simulink model "extTorqueObserver"  (R2017b)
settings: Solver=VariableStepAuto  StartTime=0.0  StopTime=10.0  RelTol=1e-3
undefined symbols (not defined in the file): D, Denv, F, g_reac, I, J_inv, Jmn, Jn, Kenv, Kt, Ktn, M, s, tau_g, tau_int
settings Model: Creator=dinies33  LastModifiedBy=dinies33

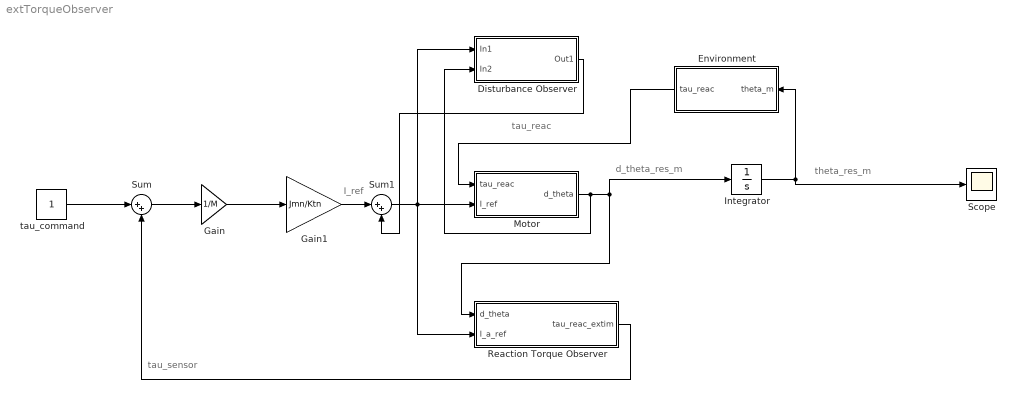
== system extTorqueObserver ==
  note: tau_sensor
  note: tau_reac
  note: theta_res_m
  note: d_theta_res_m
  note: I_ref
  Disturbance Observer : Subsystem
  Environment : Subsystem
  Gain : Gain  Gain=1/M
  Gain1 : Gain  Gain=Jmn/Ktn
  Integrator : Integrator
  Motor : Subsystem
  "Reaction Torque Observer " : Subsystem
  Scope : Scope
  Sum : Sum  Inputs=|++
  Sum1 : Sum  Inputs=|++
  "tau_command " : Constant
  wires:
  Sum/1 -> Gain/1
  Gain/1 -> Gain1/1
  Gain1/1 -> Sum1/1
  Sum1/1 -> Disturbance Observer/1(In1), Motor/2(I_ref), "Reaction Torque Observer "/2("I_a_ref ")
  Motor/1("d_theta ") -> "Reaction Torque Observer "/1("d_theta "), Integrator/1, Disturbance Observer/2(In2)
  Disturbance Observer/1(Out1) -> Sum1/2
  "Reaction Torque Observer "/1("tau_reac_extim ") -> Sum/2
  Environment/1("tau_reac ") -> Motor/1(tau_reac)
  Integrator/1 -> Scope/1, Environment/1(theta_m)
  "tau_command "/1 -> Sum/1

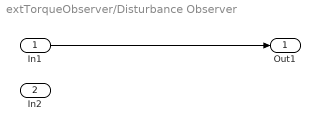
== system extTorqueObserver/Disturbance Observer ==
  In1 : Inport
  In2 : Inport  Port=2
  Out1 : Outport
  wires:
  In1/1 -> Out1/1

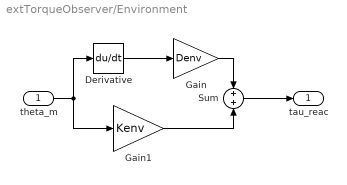
== system extTorqueObserver/Environment ==
  theta_m : Inport
  Derivative : Derivative  CoefficientInTFapproximation=1
  Gain : Gain  Gain=Denv
  Gain1 : Gain  Gain=Kenv
  Sum : Sum  Inputs=+|+
  "tau_reac " : Outport
  wires:
  Derivative/1 -> Gain/1
  Gain/1 -> Sum/1
  Sum/1 -> "tau_reac "/1
  theta_m/1 -> Gain1/1, Derivative/1
  Gain1/1 -> Sum/2

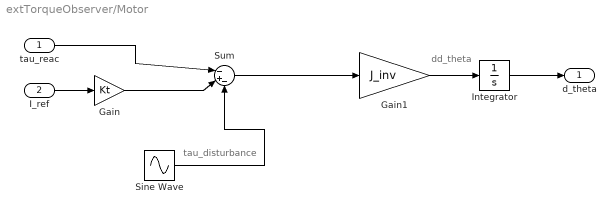
== system extTorqueObserver/Motor ==
  note: dd_theta
  note: tau_disturbance
  tau_reac : Inport
  I_ref : Inport  Port=2
  Gain : Gain  Gain=Kt
  Gain1 : Gain  Gain=J_inv
  Integrator : Integrator
  Sine Wave : Sin  SampleTime=0
  Sum : Sum  Inputs=|-+-
  "d_theta " : Outport
  wires:
  Gain/1 -> Sum/2
  Sum/1 -> Gain1/1
  I_ref/1 -> Gain/1
  tau_reac/1 -> Sum/1
  Sine Wave/1 -> Sum/3
  Gain1/1 -> Integrator/1
  Integrator/1 -> "d_theta "/1

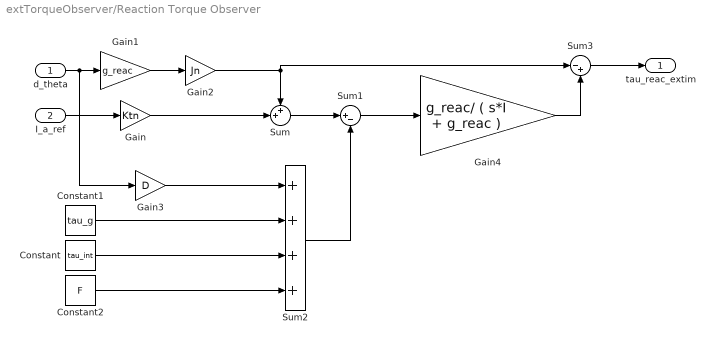
== system extTorqueObserver/Reaction Torque Observer  ==
  "d_theta " : Inport
  "I_a_ref " : Inport  Port=2
  Constant : Constant  Value=tau_int
  Constant1 : Constant  Value=tau_g
  Constant2 : Constant  Value=F
  Gain : Gain  Gain=Ktn
  Gain1 : Gain  Gain=g_reac
  Gain2 : Gain  Gain=Jn
  Gain3 : Gain  Gain=D
  Gain4 : Gain  Gain=g_reac/ ( s*I + g_reac )
  Sum : Sum  Inputs=++|
  Sum1 : Sum  Inputs=|+-
  Sum2 : Sum  Inputs=++++
  Sum3 : Sum  Inputs=|-+
  "tau_reac_extim " : Outport
  wires:
  "I_a_ref "/1 -> Gain/1
  "d_theta "/1 -> Gain3/1, Gain1/1
  Gain1/1 -> Gain2/1
  Gain/1 -> Sum/2
  Gain2/1 -> Sum3/1, Sum/1
  Sum/1 -> Sum1/1
  Sum2/1 -> Sum1/2
  Gain3/1 -> Sum2/1
  Constant1/1 -> Sum2/2
  Constant/1 -> Sum2/3
  Constant2/1 -> Sum2/4
  Sum1/1 -> Gain4/1
  Sum3/1 -> "tau_reac_extim "/1
  Gain4/1 -> Sum3/2
